simulink model "afmotor_slsp"  (Simulink 8.0)
settings: Solver=ode3  SolverMode=SingleTasking  StartTime=0.0  StopTime=10.0  RelTol=1e-3
settings Model: Creator=gcampa  LastModifiedBy=gcampa  ExtModeTrigDuration=2
settings DataIOCC: SignalLoggingSaveFormat=ModelDataLogs  SaveOutput=off  SaveTime=off
settings OptimizationCC: OptimizeModelRefInitCode=on  LifeSpan=1
settings DebuggingCC: SolverPrmCheckMsg=none  FcnCallInpInsideContextMsg=EnableAllAsWarning  StrictBusMsg=Warning
settings HardwareCC: ProdBitPerInt=16  ProdBitPerPointer=16  ProdIntDivRoundTo=Zero  ProdEndianess=LittleEndian  ProdWordSize=8  ProdHWDeviceType=Atmel->AVR
settings RTWCC: SystemTargetFile=realtime.tlc  GenerateMakefile=off  TemplateMakefile=realtime.tmf  Description=Real-Time Toolbox  RTWVerbose=off  ProcessScript=realtime_make_rtw_hook
settings STFCustomTargetCC: TargetLibSuffix=.a  CodeReplacementLibrary=ANSI_C  GenerateSampleERTMain=on  ERTCustomFileBanners=on  SupportNonInlinedSFcns=off  SupportVariableSizeSignals=on  GRTInterface=off  SystemTargetFile=realtime.tlc
settings ERTTargetCC: CodeReplacementLibrary=ANSI_C  MultiwordLength=2048  GenerateSampleERTMain=on  ParMdlRefBuildCompliant=off  CompOptLevelCompliant=off  ConcurrentExecutionCompliant=off  CombineOutputUpdateFcns=off  ERTFirstTimeCompliant=off  SupportContinuousTime=on  SupportVariableSizeSignals=on  ModelStepFunctionPrototypeControlCompliant=off  CPPClassGenCompliant=off  ExtModeTransport=3  ExtModeMexFile=ext_serial_win32_comm  ExtModeMexArgs=0 1 9600  InlinedParameterPlacement=NonHierarchical  ERTSrcFileBannerTemplate=realtime_code_template.cgt  ERTHdrFileBannerTemplate=realtime_code_template.cgt  ERTDataSrcFileTemplate=realtime_code_template.cgt  ERTDataHdrFileTemplate=realtime_code_template.cgt  ERTCustomFileTemplate=realtime_file_process.tlc  ConvertIfToSwitch=off  SuppressUnreachableDefaultCases=off
settings SettingsController: Description=Run on Hardware Dialog  TargetExtensionPlatform=Arduino Uno
settings MATStruct: Set_host_COM_port=[0.0]  COM_port_number=1  COM_port_baud_rate=115200  Enable_overrun_detection=[0.0]  Digital_output_to_set_on_overrun=13  Analog_input_reference_voltage=[0.0]  Serial0_baud_rate=9600

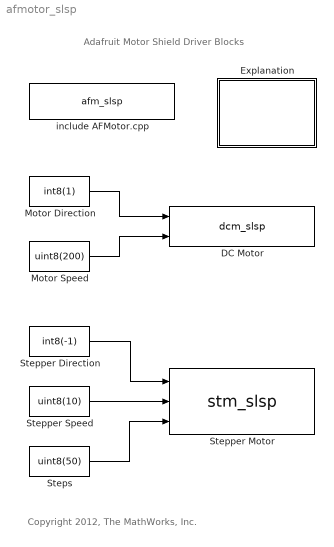
== system afmotor_slsp ==
  note: Adafruit Motor Shield Driver Blocks
  note: Copyright 2012, The MathWorks, Inc.
  DC Motor : S-Function  InitFcn=try, set_param(gcb,'FunctionName','dcm_slsp'), end  FunctionName=dcm_slsp  Parameters=uint8(4)  SFunctionModules=dcm_slsp_wrapper  WizardData=DataTag0  EnableBusSupport=off  mask(S-Function Builder){}
      mask init:
      | val = [[.9  0.75 0.75 1 1 .9 .9 1]',[1 1 0.75 0.75 .9 .9 1 .9]'];try , sys = get_param(gcb,'SfunBuilderFcnName');if isempty(sys), sys = get_param(gcb,'FunctionName'); end,catch, sys = get_param(gcb,'FunctionName'); end
      settings: CopyFcn=set_param(gcbh,'LinkStatus','none')  PreSaveFcn=try, set_param(gcb,'FunctionName','dcm_slsp'), end  OpenFcn=sfunctionwizard(gcbh)
      mask Display: plot(val(:,1),val(:,2)),disp(sys), port_label('input',1,'dir'), port_label('input',2,'spd')
  Explanation : Subsystem
      mask Display: disp('Double click \nfor explanation')
  Motor Direction : Constant  Value=int8(1)
  Motor Speed : Constant  Value=uint8(200)
  Stepper Direction : Constant  Value=int8(-1)
  Stepper Motor : S-Function  InitFcn=try, set_param(gcb,'FunctionName','stm_slsp'), end  FunctionName=stm_slsp  Parameters=uint8(1),uint8(1)  SFunctionModules=stm_slsp_wrapper  WizardData=DataTag1  EnableBusSupport=off  mask(S-Function Builder){}
      mask init: same as afmotor_slsp/DC Motor
      settings: CopyFcn=set_param(gcbh,'LinkStatus','none')  PreSaveFcn=try, set_param(gcb,'FunctionName','stm_slsp'), end  OpenFcn=sfunctionwizard(gcbh)
      mask Display: plot(val(:,1),val(:,2)),disp(sys), port_label('input',1,'dir'), port_label('input',2,'spd'), port_label('input',3,'stp')
  Stepper Speed : Constant  Value=uint8(10)
  Steps : Constant  Value=uint8(50)
  include AFMotor.cpp : S-Function  InitFcn=try, set_param(gcb,'FunctionName','afm_slsp'), end  FunctionName=afm_slsp  SFunctionModules=afm_slsp_wrapper  WizardData=DataTag2  EnableBusSupport=off  mask(S-Function Builder){}
      mask help: Simulink:masks:SFunctionBuilder_MD
      mask init: same as afmotor_slsp/DC Motor
      settings: CopyFcn=set_param(gcbh,'LinkStatus','none')  PreSaveFcn=try, set_param(gcb,'FunctionName','afm_slsp'), end  OpenFcn=sfunctionwizard(gcbh)
      mask Display:
      | plot(val(:,1),val(:,2))
      | disp(sys)
  wires:
  Stepper Direction/1 -> Stepper Motor/1
  Stepper Speed/1 -> Stepper Motor/2
  Steps/1 -> Stepper Motor/3
  Motor Direction/1 -> DC Motor/1
  Motor Speed/1 -> DC Motor/2

== system afmotor_slsp/Explanation ==
  note: GENERAL EXPLANATION:
      | --------------------------------------
      |
      | This model contains DC and Stepper Motor drivers for use with the (Arduino)
      | Adafruit Motor Shield (http://www.adafruit.com/products/81).
      |
      |
      | RUNNING THE MODEL ON THE BOARD:
      | ----------------------------------------------------------
      |
      | To run the model on an arduino board you should:
      |
      | 1) run "targetinstaller" from the MATLAB command line and install the simulink
      | support package for arduino.
      |
      | 2) In the model, go to "Tools -> Run on Target Hardware -> Prepare to Run" or
      | "Tools -> Run on Target Hardware -> Options..." to make sure that the settings
      | correspond to your version of arduino board.
      |
      | 3) download the adafruit motor library from
      | https://github.com/adafruit/Adafruit-Motor-Shield-library/zipball/master,
      | uncompress it, and place both AFMotor.h and AFMotor.cpp in the current MATLAB
      | folder where the model is.
      |
      | 4) Build the s-functions and TLC files by clicking on the "Build/Save" button of each
      | of the three the s-function builder dialog boxes.
      |
      | 5) Rename the *_wrapper.c files to *_wrapper.cpp, then open them and and add :
      | ' extern "C" ' right before the definition of the update and output functions
      | (before the void). Also see page 17 of the DriverGuide.pdf
      |  document for an explanation of why this is necessary.
      |
      | 6) Simulate the model to check that there are no errors.
      | (The model should not do anything in simulation).
      |
      | 7) Make sure the board is connected, and go to "Tools -> Run on Target Hardware
      | -> Run". This will build an arduino executable and download it on the board.
      | If the Motor Shield is mounted on the top the executable should run a DC motor
      | on port #4 and move the stepper motor connected on ports 1 and 2 every 2 seconds.
      |
      | 8) Note that every time you change a parameter in any of the s-function
      | builder blocks, steps 4 to 7 need to be redone. Also note that you need the
      |  "include AFMotor.cpp" block to be in the model
      |  when using either of the two motor driver blocks.
      |
      |
      | DC MOTOR BLOCK:
      | -----------------------------
      |
      | Every time this block is executed it sets direction and speed of a given DC motor.
      |
      | The first input is the direction (mode) of the motor (positive=forward, 0=release,
      | negative=backward), while the second input is the desired speed (0 to 255).
      | The parameter in the mask is the number of the motor (1 to 4).
      |
      |
      | STEPPER MOTOR BLOCK:
      | ---------------------------------------
      |
      | Every time this block is executed it rotates a given stepper motor by a given
      | number of steps. Execution is suspended while the motor is running and is
      | resumed when the motor completes its rotation.
      |
      | The first input is the direction (mode) of the motor (positive=forward,
      | 0=release, negative=backward), the second input is the desired speed (0 to 255),
      | and the third is the number of desired steps (0 to 255). The first parameter in the
      | mask is the number of the stepper motor (1 or 2). The second parameter is the
      | motion style (single, double, interleave, microstep).
      |
      |
      | SEE ALSO:
      | ----------------
      | Note that many of the block parameters are the same as the ones used in the
      | MATLAB Support Package for Arduino, so you might also have a look at that
      | package for additional explanations:
      | http://www.mathworks.com/matlabcentral/fileexchange/32374
